simulink model "Demo6"  (Simulink 6.5)
settings: Solver=FixedStepDiscrete  StartTime=0.0  StopTime=1  FixedStep=500e-6  RelTol=1e-3
libraries: powerlib_extras x1
settings Model: Creator=sybille  LastModifiedBy=PC_0  ExtModeAutoUpdateStatusClock=off
settings DataIOCC: SignalLoggingName=sigsOut
settings OptimizationCC: BooleanDataType=off  InlineInvariantSignals=on
settings DebuggingCC: CheckExecutionContextPreStartOutputMsg=on  CheckExecutionContextRuntimeOutputMsg=on  SolverPrmCheckMsg=none  MultiTaskDSMMsg=warning  MultiTaskCondExecSysMsg=none  StrictBusMsg=None
settings HardwareCC: TargetUnknown=on
settings RTWCC: IncludeERTFirstTime=on

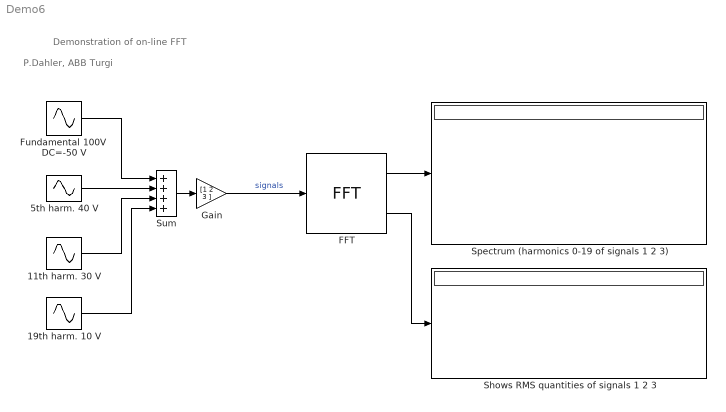
== system Demo6 ==
  note: P.Dahler, ABB Turgi
  note: Demonstration of on-line FFT
  "11th harm. 30 V " : Sin  Amplitude=30  Frequency=11*50*2*pi  SampleTime=0
  "19th harm. 10 V " : Sin  Amplitude=10  Frequency=19*50*2*pi  SampleTime=0
  "5th harm. 40 V " : Sin  Amplitude=40  Frequency=5*50*2*pi  SampleTime=0
  FFT : powerlib_extras/Discrete Measurements/FFT  DialogController=PMDialogs.PMDefaultMaskDlg  SystemSampleTime=-1  Nsig=3  f1=50  Ts=500e-6  TsFFT=0.1  base="[1 1  1   ]"  nDec=0  mask="[1 -1  1  ]"  figure_N=2
  Fundamental 100V  DC=-50 V : Sin  Amplitude=100  Bias=-50  Frequency=50*2*pi  Phase=pi/2  SampleTime=0
  Gain : Gain  Gain="[1 2  3 ]"  SaturateOnIntegerOverflow=on
  Shows RMS quantities of signals 1 2 3 : Display
      settings: Format=bank
  Spectrum (harmonics 0-19 of signals 1 2 3) : Display
      settings: Format=bank
  Sum : Sum  Inputs=++++  SaturateOnIntegerOverflow=on  InputSameDT=on
  wires:
  Fundamental 100V  DC=-50 V/1 -> Sum/1
  "5th harm. 40 V "/1 -> Sum/2
  "11th harm. 30 V "/1 -> Sum/3
  "19th harm. 10 V "/1 -> Sum/4
  FFT/2 -> Shows RMS quantities of signals 1 2 3/1
  FFT/1 -> Spectrum (harmonics 0-19 of signals 1 2 3)/1
  Gain/1 -> FFT/1  "signals"
  Sum/1 -> Gain/1
